simulink model "winter_simulink_IMM_control_2states"  (R2022a)
settings: Solver=FixedStepAuto  StartTime=0  StopTime=stop_time  FixedStep=simulation.time_step_H
values from neighbouring files (symbols this model uses):
  B_eq = param{6}    [measurement.m]    (also in measurement_2states.m; measurement_2states_3mes.m; measurement_3measure.m)
  rho = param{2}    [measurement_3measure.m]
undefined symbols (not defined in the file or in its folder): blade, dt, Gc, gearbox, generator, I_eq, IMM, lambda_vector, lookup_cP, omega_rated, pitch_range, pitch_vector, rotor, simulation, stop_time, T_R0, wind
libraries: simulink x2
settings Model: Creator=Niccolò  LastModifiedBy=Niccolò
settings SolverCC: ZeroCrossAlgorithm=Adaptive
settings DebuggingCC: IgnoredZcDiagnostic=none

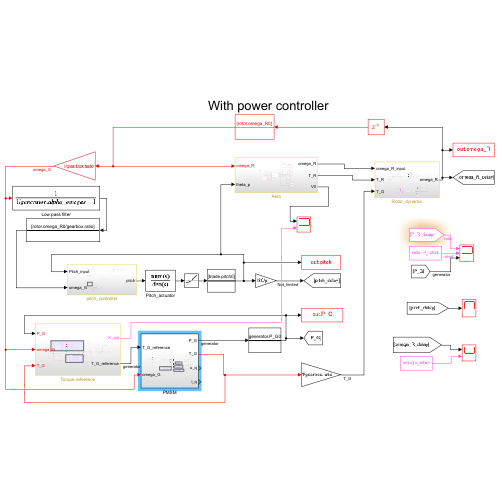
[thumbnail: Simulink's stored preview of the top-level diagram]
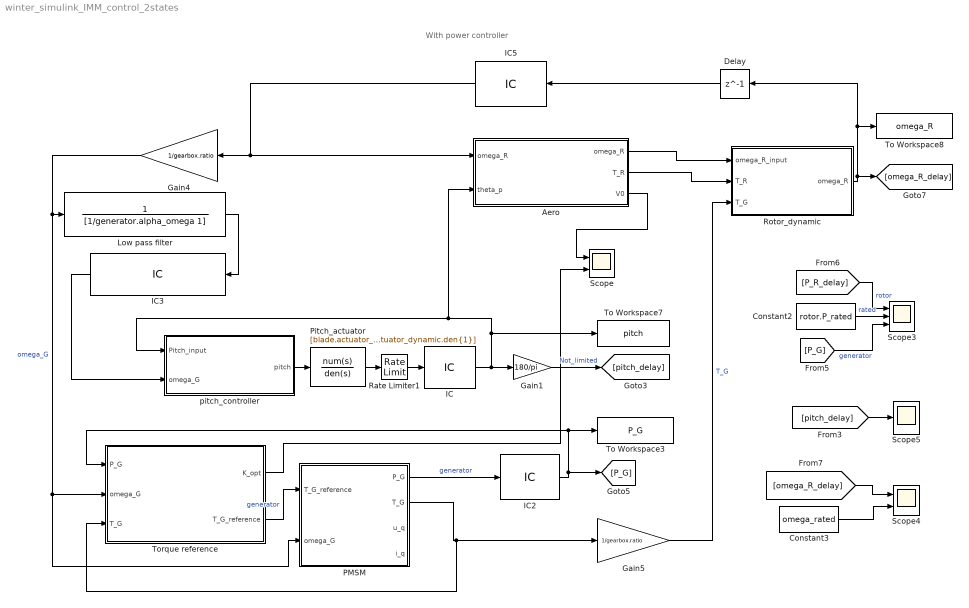
== system winter_simulink_IMM_control_2states ==
  note: With power controller
  Aero : Subsystem
  Constant2 : Constant  Value=rotor.P_rated
  Constant3 : Constant  Value=omega_rated
  Delay : Delay  DelayLength=1  InitialCondition=rotor.omega_R0
  Gain1 : Gain  Gain=180/pi
  Gain4 : Gain  Gain=1/gearbox.ratio
  Gain5 : Gain  Gain=1/gearbox.ratio
  IC : InitialCondition  Value=blade.pitch0
  IC2 : InitialCondition  Value=generator.P_G0
  IC3 : InitialCondition  Value=rotor.omega_R0/gearbox.ratio
  IC5 : InitialCondition  Value=rotor.omega_R0
  Low pass filter : TransferFcn  Denominator=[1/generator.alpha_omega 1]
  PMSM : Subsystem
  Pitch_actuator : TransferFcn  Numerator=[blade.actuator_dynamic.num{1}]  Denominator=[blade.actuator_dynamic.den{1}]
  Rate Limiter1 : RateLimiter  RisingSlewLimit=blade.pitch_rate  FallingSlewLimit=-blade.pitch_rate  SampleTimeMode=inherited
  Rotor_dynamic : Subsystem
  Scope : Scope  NumInputPorts=2
  Scope3 : Scope  NumInputPorts=3
  Scope4 : Scope  NumInputPorts=2
  Scope5 : Scope
  To Workspace3 : ToWorkspace  VariableName=P_G  SaveFormat=Timeseries  SampleTime=-1
  To Workspace7 : ToWorkspace  VariableName=pitch  SaveFormat=Timeseries  SampleTime=-1
  To Workspace8 : ToWorkspace  VariableName=omega_R  SaveFormat=Timeseries  SampleTime=-1
  Torque reference : Subsystem
  pitch_controller : Subsystem
  wires:
  [pitch_delay] -> Scope5/1
  Gain4/1 -> Low pass filter/1, PMSM/2(omega_G), Torque reference/2(omega_G)  "omega_G"
  Rate Limiter1/1 -> IC/1
  [P_R_delay] -> Scope3/1  "rotor"
  Constant3/1 -> Scope4/2
  Constant2/1 -> Scope3/2  "rated"
  [omega_R_delay] -> Scope4/1
  Gain1/1 -> [pitch_delay]  "Not_limited"
  [P_G] -> Scope3/3  "generator"
  Torque reference/2(T_G_reference) -> PMSM/1(T_G_reference)  "generator"
  pitch_controller/1(pitch) -> Pitch_actuator/1
  Pitch_actuator/1 -> Rate Limiter1/1
  Gain5/1 -> Rotor_dynamic/3(T_G)  "T_G"
  IC/1 -> Gain1/1, To Workspace7/1, pitch_controller/1(Pitch_input), Aero/2(theta_p)
  IC3/1 -> pitch_controller/2(omega_G)
  Rotor_dynamic/1(omega_R) -> Delay/1, To Workspace8/1, [omega_R_delay]
  IC5/1 -> Aero/1("omega_R "), Gain4/1
  IC2/1 -> [P_G], Torque reference/1(P_G), To Workspace3/1
  Aero/1(omega_R) -> Rotor_dynamic/1(omega_R_input)
  Aero/2(T_R) -> Rotor_dynamic/2(T_R)
  Low pass filter/1 -> IC3/1
  Delay/1 -> IC5/1
  Aero/3(V0) -> Scope/1
  Torque reference/1(K_opt) -> Scope/2
  PMSM/2(T_G) -> Torque reference/3(T_G), Gain5/1
  PMSM/1(P_G) -> IC2/1  "generator"

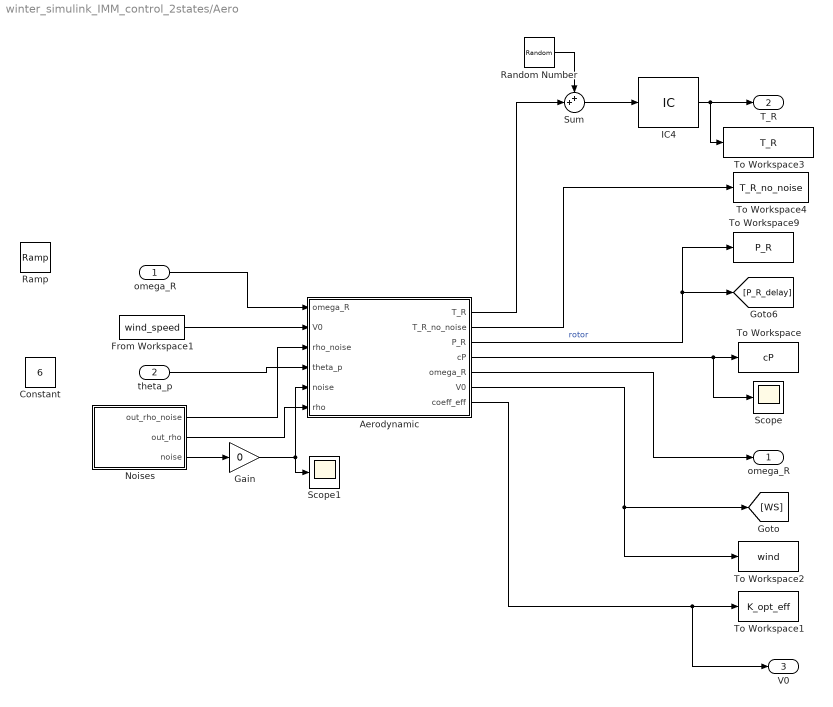
== system winter_simulink_IMM_control_2states/Aero ==
  "omega_R " : Inport
  theta_p : Inport  Port=2
  Aerodynamic : MATLAB Function  TreatAsAtomicUnit=on
  Constant : Constant  Value=6
  From Workspace1 : FromWorkspace  VariableName=wind_speed  SampleTime=1/wind.sample_f
  Gain : Gain  Gain=0
  IC4 : InitialCondition  Value=T_R0
  Noises : Subsystem
  Ramp : simulink/Sources/Ramp  slope=2/(stop_time-100)  start=100  InitialOutput=6
  Random Number : RandomNumber  Variance=IMM.Q(1)  SampleTime=simulation.time_step_H
  Scope : Scope
  Scope1 : Scope
  Sum : Sum  Inputs=++|
  To Workspace : ToWorkspace  VariableName=cP  SaveFormat=Timeseries  SampleTime=-1
  To Workspace1 : ToWorkspace  VariableName=K_opt_eff  SaveFormat=Timeseries  SampleTime=-1
  To Workspace2 : ToWorkspace  VariableName=wind  SaveFormat=Timeseries  SampleTime=-1
  To Workspace3 : ToWorkspace  VariableName=T_R  SaveFormat=Timeseries  SampleTime=-1
  To Workspace4 : ToWorkspace  VariableName=T_R_no_noise  SaveFormat=Timeseries  SampleTime=-1
  To Workspace9 : ToWorkspace  VariableName=P_R  SaveFormat=Timeseries  SampleTime=-1
  omega_R : Outport
  T_R : Outport  Port=2
  V0 : Outport  Port=3
  wires:
  "omega_R "/1 -> Aerodynamic/1("omega_R ")
  theta_p/1 -> Aerodynamic/4(theta_p)
  Aerodynamic/7(coeff_eff) -> V0/1, To Workspace1/1
  IC4/1 -> To Workspace3/1, T_R/1
  From Workspace1/1 -> Aerodynamic/2("V0 ")
  Aerodynamic/1(T_R) -> Sum/2
  Aerodynamic/2(T_R_no_noise) -> To Workspace4/1
  Aerodynamic/4(cP) -> Scope/1, To Workspace/1
  Aerodynamic/6(V0) -> To Workspace2/1, [WS]
  Aerodynamic/3(P_R) -> [P_R_delay], To Workspace9/1  "rotor"
  Noises/3(noise) -> Gain/1
  Gain/1 -> Aerodynamic/5(noise), Scope1/1
  Random Number/1 -> Sum/1
  Aerodynamic/5(omega_R) -> omega_R/1
  Sum/1 -> IC4/1
  Noises/1(out_rho_noise) -> Aerodynamic/3(rho_noise)
  Noises/2(out_rho) -> Aerodynamic/6(rho)

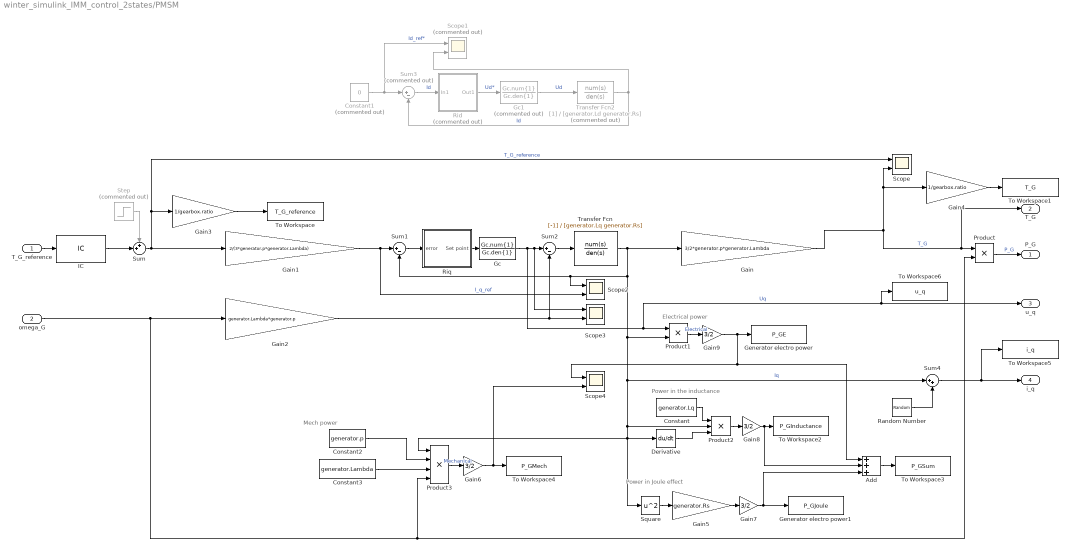
== system winter_simulink_IMM_control_2states/PMSM ==
  note: Power in Joule effect
  note: Power in the inductance
  note: Electrical power
  note: Mech power
  T_G_reference : Inport
  omega_G : Inport  Port=2
  Add : Sum  Inputs=3
  Constant : Constant  Value=generator.Lq
  Constant1 : Constant  Commented=on  Value=0
  Constant2 : Constant  Value=generator.p
  Constant3 : Constant  Value=generator.Lambda
  Derivative : Derivative
  Gain : Gain  Gain=3/2*generator.p*generator.Lambda
  Gain1 : Gain  Gain=2/(3*generator.p*generator.Lambda)
  Gain2 : Gain  Gain=generator.Lambda*generator.p
  Gain3 : Gain  Gain=1/gearbox.ratio
  Gain4 : Gain  Gain=1/gearbox.ratio
  Gain5 : Gain  Gain=generator.Rs
  Gain{6..9} (4 alike) : Gain  Gain=3/2
  Gc : TransferFcn  Numerator=Gc.num{1}  Denominator=Gc.den{1}
  Gc1 : TransferFcn  Commented=on  Numerator=Gc.num{1}  Denominator=Gc.den{1}
  Generator electro power : ToWorkspace  VariableName=P_GE  SaveFormat=Timeseries  SampleTime=-1
  Generator electro power1 : ToWorkspace  VariableName=P_GJoule  SaveFormat=Timeseries  SampleTime=-1
  IC : InitialCondition  Value=generator.T_G0
  Product : Product
  Product1 : Product
  Product2 : Product  Inputs=3
  Product3 : Product  Inputs=4
  Random Number : RandomNumber  Variance=IMM.Q(2,2)  SampleTime=simulation.time_step_H
  Rid : Subsystem  Commented=on
  Riq : Subsystem
  Scope{,2..4} (4 alike) : Scope  NumInputPorts=2
  Scope1 : Scope  Commented=on  NumInputPorts=2
  Square : Math  Operator=square
  Step : Step  Commented=on  Time=0.5  SampleTime=0
  Sum : Sum  Inputs=++|
  Sum1 : Sum  Inputs=|+-
  Sum2 : Sum  Inputs=|+-
  Sum3 : Sum  Commented=on  Inputs=|+-
  Sum4 : Sum  Inputs=|++
  To Workspace : ToWorkspace  VariableName=T_G_reference  SaveFormat=Timeseries  SampleTime=-1
  To Workspace1 : ToWorkspace  VariableName=T_G  SaveFormat=Timeseries  SampleTime=-1
  To Workspace2 : ToWorkspace  VariableName=P_GInductance  SaveFormat=Timeseries  SampleTime=-1
  To Workspace3 : ToWorkspace  VariableName=P_GSum  SaveFormat=Timeseries  SampleTime=-1
  To Workspace4 : ToWorkspace  VariableName=P_GMech  SaveFormat=Timeseries  SampleTime=-1
  To Workspace5 : ToWorkspace  VariableName=i_q  SaveFormat=Timeseries  SampleTime=-1
  To Workspace6 : ToWorkspace  VariableName=u_q  SaveFormat=Timeseries  SampleTime=-1
  Transfer Fcn : TransferFcn  Numerator=[-1]  Denominator=[generator.Lq generator.Rs]
  Transfer Fcn2 : TransferFcn  Commented=on  Denominator=[generator.Ld generator.Rs]
  P_G : Outport
  T_G : Outport  Port=2
  u_q : Outport  Port=3
  i_q : Outport  Port=4
  wires:
  Gc/1 -> To Workspace6/1, u_q/1, Product1/1, Scope3/1, Sum2/1  "Uq"
  Gain/1 -> T_G/1, Product/1, Gain4/1, Scope/2  "T_G"
  Riq/1(Set point) -> Gc/1
  Sum1/1 -> Riq/1(error)
  Transfer Fcn/1 -> Gain/1, Scope2/1, Sum1/2, Product1/2, Sum4/1, Product3/1, Square/1, Derivative/1, Product2/2  "Iq"
  Product/1 -> P_G/1  "P_G"
  Gain1/1 -> Scope2/2, Sum1/1  "I_q_ref"
  Sum/1 -> Gain1/1, Scope/1, Gain3/1  "T_G_reference"
  T_G_reference/1 -> IC/1
  Step/1 -> Sum/1
  Sum2/1 -> Transfer Fcn/1
  Gain3/1 -> To Workspace/1
  IC/1 -> Sum/2
  Gain5/1 -> Gain7/1
  Square/1 -> Gain5/1
  Derivative/1 -> Product2/3
  Constant/1 -> Product2/1
  Product2/1 -> Gain8/1
  Gc1/1 -> Transfer Fcn2/1  "Ud"
  Rid/1(Out1) -> Gc1/1  "Ud*"
  Transfer Fcn2/1 -> Sum3/2, Scope1/2  "Id"
  Constant1/1 -> Scope1/1, Sum3/1  "Id_ref*"
  Sum3/1 -> Rid/1(In1)  "Id"
  Add/1 -> To Workspace3/1
  Constant2/1 -> Product3/2
  Constant3/1 -> Product3/3
  Product3/1 -> Gain6/1  "Mechanical"
  Product1/1 -> Gain9/1  "Electrical"
  Gain2/1 -> Scope3/2, Sum2/2
  omega_G/1 -> Product/2, Product3/4, Gain2/1
  Gain6/1 -> Scope4/2, To Workspace4/1
  Gain7/1 -> Generator electro power1/1, Add/3
  Gain8/1 -> To Workspace2/1, Add/2
  Gain9/1 -> Generator electro power/1, Add/1, Scope4/1
  Gain4/1 -> To Workspace1/1
  Sum4/1 -> i_q/1, To Workspace5/1
  Random Number/1 -> Sum4/2

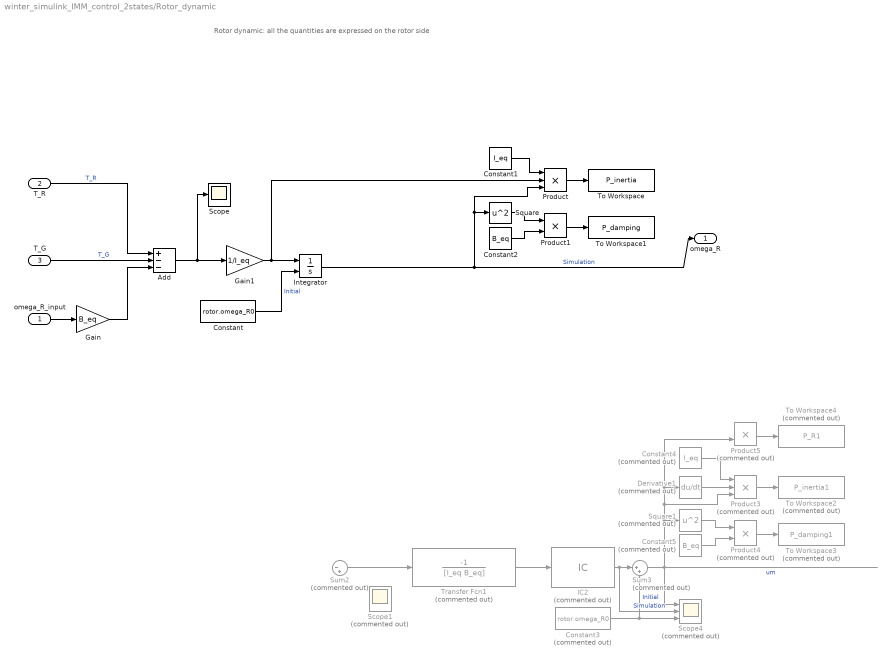
== system winter_simulink_IMM_control_2states/Rotor_dynamic ==
  note: Rotor dynamic: all the quantities are expressed on the rotor side
  omega_R_input : Inport
  T_R : Inport  Port=2
  T_G : Inport  Port=3
  Add : Sum  Inputs=+--
  Constant : Constant  Value=rotor.omega_R0
  Constant1 : Constant  Value=I_eq
  Constant2 : Constant  Value=B_eq
  Constant3 : Constant  Commented=on  Value=rotor.omega_R0
  Constant4 : Constant  Commented=on  Value=I_eq
  Constant5 : Constant  Commented=on  Value=B_eq
  Derivative1 : Derivative  Commented=on
  Gain : Gain  Gain=B_eq
  Gain1 : Gain  Gain=1/I_eq
  IC2 : InitialCondition  Commented=on  Value=rotor.omega_R0
  Integrator : Integrator  InitialConditionSource=external
  Product : Product  Inputs=3
  Product1 : Product
  Product3 : Product  Commented=on  Inputs=3
  Product4 : Product  Commented=on
  Product5 : Product  Commented=on
  Scope : Scope
  Scope1 : Scope  Commented=on  NumInputPorts=2
  Scope4 : Scope  Commented=on  NumInputPorts=3
  Square : Math  Operator=square
  Square1 : Math  Commented=on  Operator=square
  Sum2 : Sum  Commented=on  Inputs=|-+
  Sum3 : Sum  Commented=on  Inputs=|++
  To Workspace : ToWorkspace  VariableName=P_inertia  SaveFormat=Timeseries  SampleTime=-1
  To Workspace1 : ToWorkspace  VariableName=P_damping  SaveFormat=Timeseries  SampleTime=-1
  To Workspace2 : ToWorkspace  Commented=on  VariableName=P_inertia1  SaveFormat=Timeseries  SampleTime=-1
  To Workspace3 : ToWorkspace  Commented=on  VariableName=P_damping1  SaveFormat=Timeseries  SampleTime=-1
  To Workspace4 : ToWorkspace  Commented=on  VariableName=P_R1  SaveFormat=Timeseries  SampleTime=-1
  Transfer Fcn1 : TransferFcn  Commented=on  Numerator=[-1]  Denominator=[I_eq B_eq]
  omega_R : Outport
  wires:
  Integrator/1 -> Product/3, Square/1, omega_R/1  "Simulation"
  T_G/1 -> Add/2  "T_G"
  Constant/1 -> Integrator/2  "Initial"
  T_R/1 -> Add/1  "T_R"
  Add/1 -> Scope/1, Gain1/1
  Constant1/1 -> Product/1
  Product/1 -> To Workspace/1
  Constant2/1 -> Product1/2
  Product1/1 -> To Workspace1/1
  Square/1 -> Product1/1
  Square1/1 -> Product4/1
  Product5/1 -> To Workspace4/1
  Derivative1/1 -> Product3/2
  Product4/1 -> To Workspace3/1
  Constant4/1 -> Product3/1
  Constant5/1 -> Product4/2
  ? -> Scope1/2, Sum2/1, Product5/1  "T_R"
  ? -> Scope1/1, Sum2/2  "T_G"
  IC2/1 -> Scope4/2, Sum3/1  "Simulation"
  Sum2/1 -> Transfer Fcn1/1
  Product3/1 -> To Workspace2/1
  Transfer Fcn1/1 -> IC2/1
  Sum3/1 -> Product5/2, Derivative1/1, Product3/3, Square1/1, Scope4/1  "um"
  Constant3/1 -> Scope4/3, Sum3/2  "Initial"
  omega_R_input/1 -> Gain/1
  Gain/1 -> Add/3
  Gain1/1 -> Product/2, Integrator/1

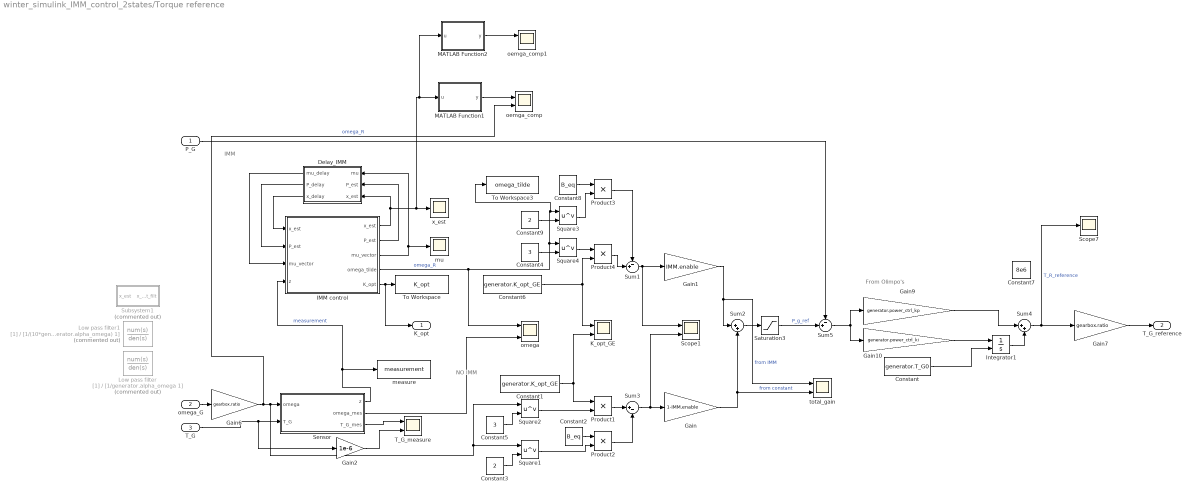
== system winter_simulink_IMM_control_2states/Torque reference ==
  note: IMM
  note: NO IMM
  note: From Olimpo's
  P_G : Inport
  omega_G : Inport  Port=2
  T_G : Inport  Port=3
  Constant : Constant  Value=generator.T_G0
  Constant1 : Constant  Value=generator.K_opt_GE
  Constant2 : Constant  Value=B_eq
  Constant3 : Constant  Value=2
  Constant4 : Constant  Value=3
  Constant5 : Constant  Value=3
  Constant6 : Constant  Value=generator.K_opt_GE
  Constant7 : Constant  Value=8e6
  Constant8 : Constant  Value=B_eq
  Constant9 : Constant  Value=2
  Delay_IMM : Subsystem
  Gain : Gain  Gain=1-IMM.enable
  Gain1 : Gain  Gain=IMM.enable
  Gain10 : Gain  Gain=generator.power_ctrl_ki
  Gain2 : Gain  Gain=1e-6
  Gain6 : Gain  Gain=gearbox.ratio
  Gain7 : Gain  Gain=gearbox.ratio
  Gain9 : Gain  Gain=generator.power_ctrl_kp
  IMM control : MATLAB Function  TreatAsAtomicUnit=on
  Integrator1 : Integrator  InitialConditionSource=external
  K_opt_GE : Scope  NumInputPorts=2
  Low pass filter : TransferFcn  Commented=on  Denominator=[1/generator.alpha_omega 1]
  Low pass filter1 : TransferFcn  Commented=on  Denominator=[1/(10*generator.alpha_omega) 1]
  MATLAB Function1 : MATLAB Function  TreatAsAtomicUnit=on
  MATLAB Function2 : MATLAB Function  TreatAsAtomicUnit=on
  Product{1..4} (4 alike) : Product
  Saturation3 : Saturate  UpperLimit=generator.P_rated  LowerLimit=0
  Scope1 : Scope  NumInputPorts=2
  Scope7 : Scope
  Sensor : MATLAB Function  TreatAsAtomicUnit=on
  Square{1..4} (4 alike) : Math  Operator=pow
  Subsystem1 : Subsystem  Commented=on
  Sum1 : Sum  Inputs=-+|
  Sum2 : Sum  Inputs=|++
  Sum3 : Sum  Inputs=|+-
  Sum4 : Sum  Inputs=|++
  Sum5 : Sum  Inputs=-+|
  T_G_measure : Scope  NumInputPorts=2
  To Workspace : ToWorkspace  VariableName=K_opt  SaveFormat=Timeseries  SampleTime=-1
  To Workspace3 : ToWorkspace  VariableName=omega_tilde  SaveFormat=Timeseries  SampleTime=-1
  measure : ToWorkspace  VariableName=measurement  SaveFormat=Timeseries  SampleTime=-1
  mu : Scope
  oemga_comp : Scope  NumInputPorts=2
  oemga_comp1 : Scope  NumInputPorts=2
  omega : Scope  NumInputPorts=3
  total_gain : Scope  NumInputPorts=2
  x_est : Scope
  K_opt : Outport
  T_G_reference : Outport  Port=2
  wires:
  Square2/1 -> Product1/2
  Gain9/1 -> Sum4/1
  Gain10/1 -> Integrator1/1
  Constant/1 -> Integrator1/2
  Sum4/1 -> Scope7/1, Gain7/1  "T_R_reference"
  Constant5/1 -> Square2/2
  Saturation3/1 -> Sum5/2  "P_g_ref"
  Integrator1/1 -> Sum4/2
  Sum5/1 -> Gain9/1, Gain10/1
  Gain7/1 -> T_G_reference/1
  P_G/1 -> Sum5/1
  IMM control/2(P_est) -> Delay_IMM/2(P_est)
  Delay_IMM/3(x_delay) -> IMM control/1("x_est ")
  Delay_IMM/2(P_delay) -> IMM control/2("P_est ")
  Delay_IMM/1(mu_delay) -> IMM control/3("mu_vector ")
  IMM control/3(mu_vector) -> Delay_IMM/1(mu), mu/1
  Constant8/1 -> Product3/1
  Square3/1 -> Product3/2
  Product4/1 -> Sum1/2
  Sum1/1 -> Scope1/1, Gain1/1
  Constant9/1 -> Square3/2
  Gain/1 -> total_gain/2, Sum2/2  "from constant"
  Sum2/1 -> Saturation3/1
  Constant3/1 -> Square1/2
  Sum3/1 -> Scope1/2, Gain/1
  Product1/1 -> Sum3/1
  Square1/1 -> Product2/2
  Product2/1 -> Sum3/2
  Constant2/1 -> Product2/1
  Gain1/1 -> total_gain/1, Sum2/1  "from IMM"
  Square4/1 -> Product4/1
  Product3/1 -> Sum1/1
  Constant1/1 -> Product1/1, K_opt_GE/2
  IMM control/5(K_opt) -> K_opt/1, To Workspace/1
  Constant4/1 -> Square4/2
  omega_G/1 -> Gain6/1
  Constant6/1 -> K_opt_GE/1, Product4/2
  Sensor/1(z) -> measure/1, IMM control/4(z)  "measurement"
  MATLAB Function1/1(y) -> oemga_comp/1
  Gain6/1 -> Square2/1, Square1/1, Sensor/1(omega), oemga_comp/2  "omega_R"
  T_G/1 -> Gain2/1, Sensor/2(T_G)
  IMM control/4(omega_tilde) -> To Workspace3/1, Square3/1, Square4/1, omega/1  "omega_R"
  Sensor/3(T_G_mes) -> T_G_measure/1
  Gain2/1 -> T_G_measure/2
  Sensor/2(omega_mes) -> omega/3
  IMM control/1(x_est) -> MATLAB Function2/1(u), MATLAB Function1/1(u), x_est/1, Delay_IMM/3(x_est)
  MATLAB Function2/1(y) -> oemga_comp1/1
  ? -> oemga_comp1/2  "omega_R"

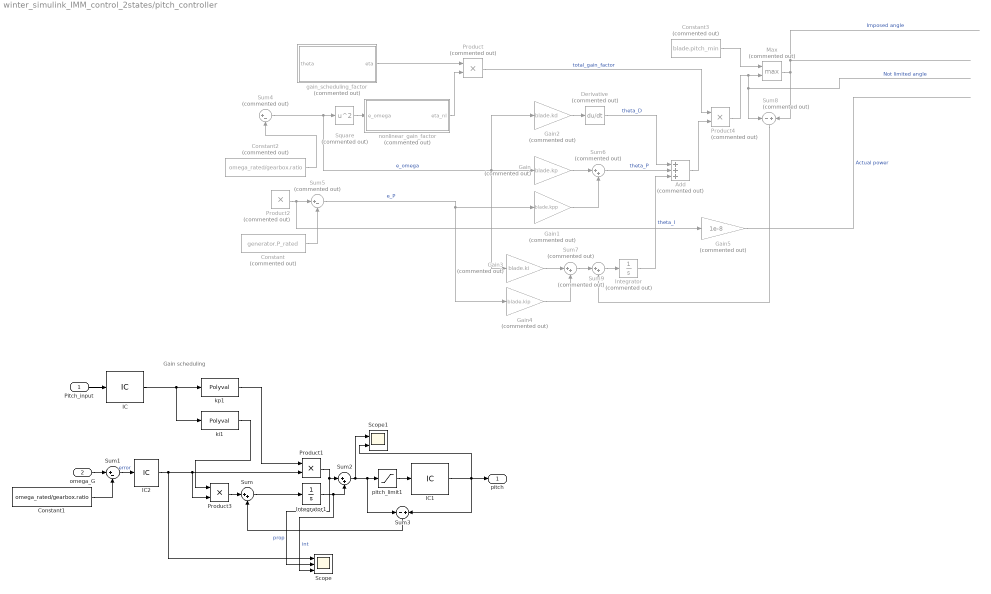
== system winter_simulink_IMM_control_2states/pitch_controller ==
  note: Gain scheduling
  Pitch_input : Inport
  omega_G : Inport  Port=2
  Add : Sum  Commented=on  Inputs=+++
  Constant : Constant  Commented=on  Value=generator.P_rated
  Constant1 : Constant  Value=omega_rated/gearbox.ratio
  Constant2 : Constant  Commented=on  Value=omega_rated/gearbox.ratio
  Constant3 : Constant  Commented=on  Value=blade.pitch_min
  Derivative : Derivative  Commented=on
  Gain : Gain  Commented=on  Gain=blade.kp
  Gain1 : Gain  Commented=on  Gain=blade.kpp
  Gain2 : Gain  Commented=on  Gain=blade.kd
  Gain3 : Gain  Commented=on  Gain=blade.ki
  Gain4 : Gain  Commented=on  Gain=blade.kip
  Gain5 : Gain  Commented=on  Gain=1e-8
  IC : InitialCondition  Value=blade.pitch0
  IC1 : InitialCondition  Value=blade.pitch0
  IC2 : InitialCondition  Value=(rotor.omega_R0 - omega_rated)/gearbox.ratio
  Integrator : Integrator  Commented=on
  Integrator1 : Integrator
  Max : MinMax  Commented=on  Function=max  Inputs=2
  Product : Product  Commented=on
  Product1 : Product
  Product2 : Product  Commented=on
  Product3 : Product
  Product4 : Product  Commented=on
  Scope : Scope  NumInputPorts=3
  Scope1 : Scope  NumInputPorts=2
  Square : Math  Commented=on  Operator=square
  Sum : Sum  Inputs=|++
  Sum1 : Sum  Inputs=|+-
  Sum2 : Sum  Inputs=|++
  Sum3 : Sum  Inputs=-|+
  Sum4 : Sum  Commented=on  Inputs=|+-
  Sum5 : Sum  Commented=on  Inputs=|+-
  Sum6 : Sum  Commented=on  Inputs=|++
  Sum7 : Sum  Commented=on  Inputs=|++
  Sum8 : Sum  Commented=on  Inputs=-|+
  Sum9 : Sum  Commented=on  Inputs=|++
  gain_scheduling_factor : MATLAB Function  Commented=on  TreatAsAtomicUnit=on
  ki1 : Polyval  Coefs=blade.ki_schedule
  kp1 : Polyval  Coefs=blade.kp_schedule
  nonlinear_gain_factor : MATLAB Function  Commented=on  TreatAsAtomicUnit=on
  pitch_limit1 : Saturate  UpperLimit=pitch_range(2)  LowerLimit=0
  pitch : Outport
  wires:
  Sum/1 -> Integrator1/1
  Constant1/1 -> Sum1/2
  Product3/1 -> Sum/1
  omega_G/1 -> Sum1/1
  ki1/1 -> Product3/1
  kp1/1 -> Product1/1
  Sum1/1 -> IC2/1  "error"
  Product1/1 -> Scope/2, Sum2/1  "prop"
  Integrator1/1 -> Scope/3, Sum2/2  "int"
  ? -> ?  "Actual value"
  Sum8/1 -> Sum9/2
  Product4/1 -> Max/2, Sum8/1  "Not limited angle"
  Add/1 -> Product4/2
  Gain4/1 -> Sum7/2
  Product2/1 -> Gain5/1, Sum5/1
  Integrator/1 -> Add/3  "theta_I"
  ? -> Product2/2
  Derivative/1 -> Add/1  "theta_D"
  Product/1 -> Product4/1  "total_gain_factor"
  Sum6/1 -> Add/2  "theta_P"
  nonlinear_gain_factor/1(eta_nl) -> Product/2
  gain_scheduling_factor/1(eta) -> Product/1
  Gain/1 -> Sum6/1
  Max/1 -> Sum8/2  "Imposed angle"
  Sum5/1 -> Gain4/1, Gain1/1  "e_P"
  ? -> Sum4/1, Product2/1
  Constant2/1 -> Sum4/2
  Sum4/1 -> Gain3/1, Gain2/1, Gain/1, Square/1  "e_omega"
  Gain2/1 -> Derivative/1
  ? -> gain_scheduling_factor/1(theta)
  Gain5/1 -> ?  "Actual power"
  Constant/1 -> Sum5/2
  Constant3/1 -> Max/1
  Sum9/1 -> Integrator/1
  Gain1/1 -> Sum6/2
  Sum7/1 -> Sum9/1
  Square/1 -> nonlinear_gain_factor/1(e_omega)
  Gain3/1 -> Sum7/1
  Pitch_input/1 -> IC/1
  Sum2/1 -> pitch_limit1/1, Sum3/1, Scope1/1
  Sum3/1 -> Sum/2
  pitch_limit1/1 -> IC1/1
  IC/1 -> ki1/1, kp1/1
  IC1/1 -> Scope1/2, pitch/1, Sum3/2
  IC2/1 -> Scope/1, Product3/2, Product1/2

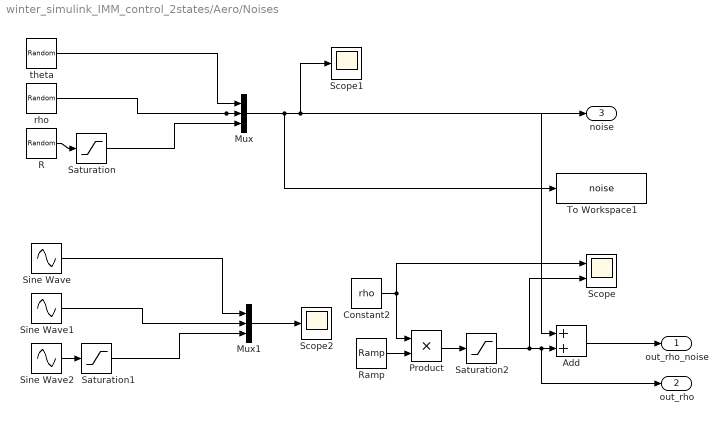
== system winter_simulink_IMM_control_2states/Aero/Noises ==
  Add : Sum
  Constant2 : Constant  Value=rho
  Mux : Mux  Inputs=3
  Mux1 : Mux  Inputs=3
  Product : Product
  R : RandomNumber  Variance=(IMM.sigma_R)^2  SampleTime=simulation.time_step_H
  Ramp : simulink/Sources/Ramp  slope=0.4/(stop_time-50)  start=50  InitialOutput=0.8
  Saturation : Saturate  UpperLimit=0  LowerLimit=-10
  Saturation1 : Saturate  UpperLimit=0  LowerLimit=-10
  Saturation2 : Saturate  UpperLimit=1.2*rho
  Scope : Scope  NumInputPorts=2
  Scope1 : Scope
  Scope2 : Scope
  Sine Wave : Sin  Amplitude=IMM.sigma_theta  Frequency=IMM.freq_theta  Phase=IMM.phase_theta  SampleTime=simulation.time_step_H
  Sine Wave1 : Sin  Amplitude=IMM.sigma_rho  Frequency=IMM.freq_rho  Phase=IMM.phase_rho  SampleTime=simulation.time_step_H
  Sine Wave2 : Sin  Amplitude=IMM.sigma_R  Frequency=IMM.freq_R  Phase=IMM.phase_R  SampleTime=simulation.time_step_H
  To Workspace1 : ToWorkspace  VariableName=noise  SaveFormat=Timeseries  SampleTime=-1
  rho : RandomNumber  Variance=(IMM.sigma_rho)^2  SampleTime=simulation.time_step_H
  theta : RandomNumber  Variance=(IMM.sigma_theta)^2  SampleTime=simulation.time_step_H
  out_rho_noise : Outport
  out_rho : Outport  Port=2
  noise : Outport  Port=3
  wires:
  Mux/1 -> To Workspace1/1, noise/1, Scope1/1
  theta/1 -> Mux/1
  rho/1 -> Add/1, Mux/2
  Saturation/1 -> Mux/3
  R/1 -> Saturation/1
  Mux1/1 -> Scope2/1
  Sine Wave2/1 -> Saturation1/1
  Sine Wave/1 -> Mux1/1
  Saturation1/1 -> Mux1/3
  Sine Wave1/1 -> Mux1/2
  Constant2/1 -> Product/1, Scope/1
  Product/1 -> Saturation2/1
  Add/1 -> out_rho_noise/1
  Saturation2/1 -> Scope/2, out_rho/1, Add/2
  Ramp/1 -> Product/2

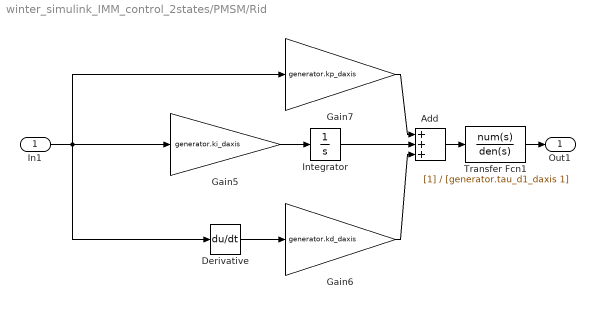
== system winter_simulink_IMM_control_2states/PMSM/Rid ==
  In1 : Inport
  Add : Sum  Inputs=+++
  Derivative : Derivative
  Gain5 : Gain  Gain=generator.ki_daxis
  Gain6 : Gain  Gain=generator.kd_daxis
  Gain7 : Gain  Gain=generator.kp_daxis
  Integrator : Integrator
  Transfer Fcn1 : TransferFcn  Denominator=[generator.tau_d1_daxis 1]
  Out1 : Outport
  wires:
  Integrator/1 -> Add/2
  Add/1 -> Transfer Fcn1/1
  Gain7/1 -> Add/1
  Gain6/1 -> Add/3
  Derivative/1 -> Gain6/1
  In1/1 -> Derivative/1, Gain7/1, Gain5/1
  Transfer Fcn1/1 -> Out1/1
  Gain5/1 -> Integrator/1

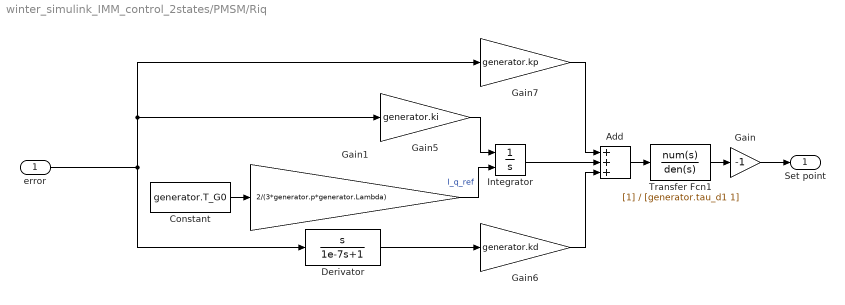
== system winter_simulink_IMM_control_2states/PMSM/Riq ==
  error : Inport
  Add : Sum  Inputs=+++
  Constant : Constant  Value=generator.T_G0
  Derivator : TransferFcn  Numerator=[1 0]  Denominator=[1e-7 1]
  Gain : Gain  Gain=-1
  Gain1 : Gain  Gain=2/(3*generator.p*generator.Lambda)
  Gain5 : Gain  Gain=generator.ki
  Gain6 : Gain  Gain=generator.kd
  Gain7 : Gain  Gain=generator.kp
  Integrator : Integrator  InitialConditionSource=external
  Transfer Fcn1 : TransferFcn  Denominator=[generator.tau_d1 1]
  Set point : Outport
  wires:
  Integrator/1 -> Add/2
  Add/1 -> Transfer Fcn1/1
  Constant/1 -> Gain1/1
  Gain7/1 -> Add/1
  Gain6/1 -> Add/3
  Derivator/1 -> Gain6/1
  Transfer Fcn1/1 -> Gain/1
  Gain5/1 -> Integrator/1
  Gain1/1 -> Integrator/2  "I_q_ref"
  Gain/1 -> Set point/1
  error/1 -> Gain5/1, Gain7/1, Derivator/1

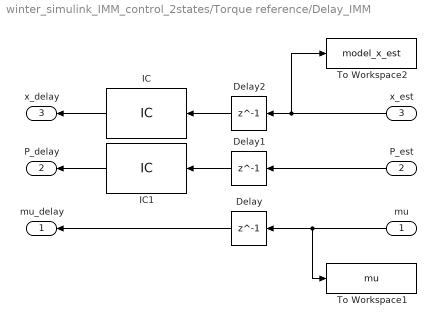
== system winter_simulink_IMM_control_2states/Torque reference/Delay_IMM ==
  mu : Inport
  P_est : Inport  Port=2
  x_est : Inport  Port=3
  Delay : Delay  DelayLength=1  InitialCondition=ones(IMM.n_models, 1)/IMM.n_models
  Delay1 : Delay  DelayLength=1  InitialCondition=IMM.P_est_initial
  Delay2 : Delay  DelayLength=1  InitialCondition=IMM.x_est_initial
  IC : InitialCondition  Value=IMM.x_est_initial
  IC1 : InitialCondition  Value=IMM.P_est_initial
  To Workspace1 : ToWorkspace  VariableName=mu  SaveFormat=Timeseries  SampleTime=-1
  To Workspace2 : ToWorkspace  VariableName=model_x_est  SaveFormat=Timeseries  SampleTime=-1
  mu_delay : Outport
  P_delay : Outport  Port=2
  x_delay : Outport  Port=3
  wires:
  Delay1/1 -> IC1/1
  P_est/1 -> Delay1/1
  Delay2/1 -> IC/1
  mu/1 -> To Workspace1/1, Delay/1
  x_est/1 -> To Workspace2/1, Delay2/1
  IC/1 -> x_delay/1
  IC1/1 -> P_delay/1
  Delay/1 -> mu_delay/1

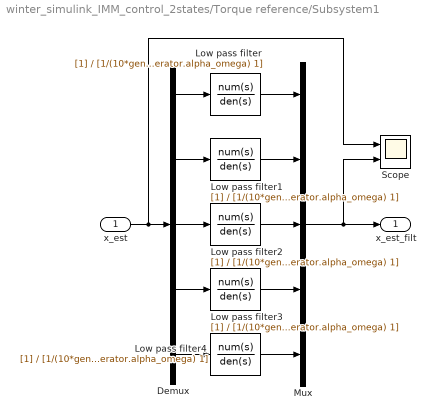
== system winter_simulink_IMM_control_2states/Torque reference/Subsystem1 ==
  x_est : Inport
  Demux : Demux  Outputs=5
  Low pass filter{,1..4} (5 alike) : TransferFcn  Denominator=[1/(10*generator.alpha_omega) 1]
  Mux : Mux  Inputs=5
  Scope : Scope  NumInputPorts=2
  x_est_filt : Outport
  wires:
  Demux/3 -> Low pass filter2/1
  Demux/1 -> Low pass filter/1
  Demux/4 -> Low pass filter3/1
  x_est/1 -> Scope/1, Demux/1
  Demux/5 -> Low pass filter4/1
  Demux/2 -> Low pass filter1/1
  Low pass filter4/1 -> Mux/5
  Low pass filter3/1 -> Mux/4
  Low pass filter2/1 -> Mux/3
  Low pass filter1/1 -> Mux/2
  Low pass filter/1 -> Mux/1
  Mux/1 -> Scope/2, x_est_filt/1

== matlab function winter_simulink_IMM_control_2states/pitch_controller/gain_scheduling_factor ==
  data: eta output; theta input; blade parameter
function eta = gain_scheduling_factor(theta, blade)

K1 = blade.K1;
K2 = blade.K2;

theta = theta*180/pi; % [deg]

eta = 1/(1+ theta/K1 + theta^2/K2);

== matlab function winter_simulink_IMM_control_2states/pitch_controller/nonlinear_gain_factor ==
  data: e_omega input; eta_nl output; blade parameter; generator parameter
function eta_nl = nonlinear_gain_factor(e_omega, blade, generator)

omega_rated = generator.omega_rated;
omega2 = omega_rated*blade.omega2omega0ratio;

eta_nl = 1 + e_omega^2/(omega2 - omega_rated)^2;

== matlab function winter_simulink_IMM_control_2states/Torque reference/MATLAB Function1 ==
  data: u input; y output
function y = fcn(u)

y = u(1,:);

== matlab function winter_simulink_IMM_control_2states/Aero/Aerodynamic ==
  data: omega_R input; V0 input; T_R output; T_R_no_noise output; P_R output; rho_noise input; theta_p input; lambda_vector parameter; pitch_vector parameter; lookup_cP parameter; cP output; rotor parameter; omega_R output; V0 output; noise input; coeff_eff output; rho input
function [T_R, T_R_no_noise, P_R, cP, omega_R, V0, coeff_eff] = Aerodynamic(omega_R, V0, rho_noise, theta_p, lambda_vector, pitch_vector, lookup_cP, rotor, noise, rho)

R = rotor.R;       % rotor radius [m]

% retrive the cP from the look-up table
lambda = omega_R*R/V0;                                                
cP = interp2(lambda_vector, pitch_vector, lookup_cP, lambda, theta_p);

P_R = 0.5*rho*V0^3*pi*R^2*cP; % rotor power [W]
T_R_no_noise = P_R/omega_R;            % rotor torque [Nm]


theta_p = theta_p + noise(1); % pitch angle [rad]
R = rotor.R + noise(3);       % rotor radius [m]

% retrive the cP from the look-up table
lambda = omega_R*R/V0;                                                
cP = interp2(lambda_vector, pitch_vector, lookup_cP, lambda, theta_p);
P_R = 0.5*rho_noise*V0^3*pi*R^2*cP; % rotor power [W]
T_R = P_R/omega_R;            % rotor torque [Nm]

coeff_eff =cP*rho*R^2; %

== matlab function winter_simulink_IMM_control_2states/Torque reference/IMM control ==
  settings: updateMethod=DISCRETE  sampleTime=simulation.time_step_H
  data: x_est output; P_est output; mu_vector output; x_est input size=[IMM.states_len, IMM.n_models]; P_est input size=[IMM.states_len, IMM.states_len, IMM.n_models]; mu_vector input size=[IMM.n_models, 1]; IMM parameter; I_eq parameter; omega_tilde output size=1; K_opt output size=1; dt parameter; z input; generator parameter; B_eq parameter
function [x_est, P_est, mu_vector, omega_tilde,  K_opt] = gain_IMM(x_est, P_est, mu_vector, IMM, I_eq, dt, z, generator, B_eq)
  % x_est -> (states_len, n_models) items containing the state estimation
  % P_est -> (states_len, states_len, n_models) containing the covariance
  
  n_models = IMM.n_models; % number of models to test
  states_len = IMM.states_len; % length of the states
  measure_len = IMM.measure_len; % length of the measurement
  Pi = IMM.Pi; 
  R = IMM.W;
  Q = IMM.Q;
  K_vector = IMM.K_vector;
  mu = zeros(n_models);
  % Vector of parameters
  param = cell(6,1);
  param{1} = I_eq; % inertia
  param{2} = 0; % cp*rho*R^2
  param{3} = generator.K_opt_GE; % K_opt
  param{4} = R; % measure noise
  param{5} = Q; % process noise 
  param{6} = B_eq; % transmission damping
 
  % Assamble the model cell
  model = cell(n_models, 1);
  for j=1:n_models
    param{2} = IMM.K_vector(j); % rho_cp_R2
    model{j} = struct('rho_cp_R2', IMM.K_vector(j), 'x_est', x_est(1:states_len, j), 'P_est', P_est(1:states_len,1:states_len,j), 'z_hat', zeros(measure_len, 1), 'P_prior', P_est(1:states_len,1:states_len,j), 'Lambda', 0, 'mu', mu_vector(j), 'mu_new', 0, 'x_tilde', zeros(states_len, 1), 'P_tilde', zeros(states_len));
  end
  
  % Filtering
  u = [0]; % input
  model = filtering(model, z, u, param, dt);
  
  % Mode probability updating
  model = probability_updating(model, z, param, dt);
  K_opt = compute_K_opt(model); % weighted mean of the filters

  % State combination
  x_est_g = zeros(states_len, 1); % global state
  [x_est_g(1:states_len, 1), ~] = state_combination(model);
  omega_tilde = x_est_g(1); % estimation of the rotational speed

  % Filter interaction
  [model, model_prob] = filter_interaction(model, Pi);
  
  % Assemble the model cell
  for j=1:n_models
    x_est(1:states_len, j) = model{j}.x_est(1:states_len);
    P_est(1:states_len,1:states_len,j) = model{j}.P_est(1:states_len, 1:states_len);
    mu_vector(j) = model{j}.mu_new(1);
  end
  
end
  
  %   _____ _  _______ 
  %  | ____| |/ /  ___|
  %  |  _| | ' /| |_   
  %  | |___| . \|  _|  
  %  |_____|_|\_\_|    
                     
  function [model] = EKF(model, z, u, param, matrices, dt)
    % y -> measurement of the rotational speed [rad/s]
    
    x_est = model.x_est;
    P_est = model.P_est;
    states_len = size(x_est, 1);
    measure_len = size(z, 1);

    F = matrices.F;
    H = matrices.H;
    Q = matrices.Q;
    R = matrices.R;
    G = matrices.G;
  
    % Prediction
    x_est = dynamic(x_est(1:states_len), u, param, dt);
    P_est = F*P_est*F' + G*Q*G';
    P_prior = P_est;
    states_len = size(x_est, 1); % number of states
  
    % Update
    [~, z_hat] = measurement(x_est, param, measure_len); % estimation of the measurement using the sensor's model
    Innovation = z - z_hat;
    S_Inno = H*P_est*H' + R;
    W = P_est*H'*inv(S_Inno); % kalman gain
    x_est = x_est + W*Innovation; % update state estimate
    P_est = (eye(states_len) - W*H)*P_est; % update covariance matrix
  
  
    model.x_est(1:states_len) = x_est(1:states_len);
    model.P_est(1:states_len, 1:states_len) = P_est(1:states_len, 1:states_len);
    model.z_hat = z_hat;
    model.P_prior = P_prior;
  end
  
  %   ____                              _      
  %  |  _ \ _   _ _ __   __ _ _ __ ___ (_) ___ 
  %  | | | | | | | '_ \ / _` | '_ ` _ \| |/ __|
  %  | |_| | |_| | | | | (_| | | | | | | | (__ 
  %  |____/ \__, |_| |_|\__,_|_| |_| |_|_|\___|
  %         |___/                              
  
  function x_new = dynamic(x_est, u, param, dt)
  
    states_len = size(x_est, 1);
    I_eq = param{1}; % Inertia
    rho_cp_R2 = param{2}; % Damping
    K_opt = param{3}; % Power coefficient
    
    omega = x_est(1);
    V0 = x_est(2);

    x_new = zeros(states_len,1);
  
    x_new(1) = omega + dt/I_eq*(1/2*pi*rho_cp_R2*V0^3/omega - K_opt*omega^2 ); % [rad/s] rotational speed
    x_new(2) = V0; % [m/s] wind speed 
  end
  

  
  %    ____                            _                         _     
  %   / ___|___  _ __ ___  _ __  _   _| |_ ___   _ __ ___   __ _| |_   
  %  | |   / _ \| '_ ` _ \| '_ \| | | | __/ _ \ | '_ ` _ \ / _` | __|  
  %  | |__| (_) | | | | | | |_) | |_| | ||  __/ | | | | | | (_| | |_ _ 
  %   \____\___/|_| |_| |_| .__/ \__,_|\__\___| |_| |_| |_|\__,_|\__(_)
  %                       |_|                                          
  
  function matrices = compute_matrices(x_est, param, dt)
  
    I_eq = param{1}; % Inertia
    rho_cp_R2 = param{2}; % Density
    K_opt = param{3}; % Power coefficient
    B_eq = param{6};
    omega = x_est(1);
    V0 = x_est(2);

    F = [1+dt/I_eq*(-1/2*rho_cp_R2*pi*V0^3/omega^2-2*K_opt*omega), (3*dt*pi*rho_cp_R2*V0^2)/(2*I_eq*omega); 0, 1];
    H = [1, 0; (-1/2*pi*rho_cp_R2*V0^3/omega^2-B_eq)*1e-6, (3/2*pi*rho_cp_R2*V0^2/omega)*1e-6];
    G = [dt/I_eq 0; 0 1];

    matrices = struct('F', F, 'H', H, 'G', G);
  end
  
  %   _____ _ _ _            _             
  %  |  ___(_) | |_ ___ _ __(_)_ __   __ _ 
  %  | |_  | | | __/ _ \ '__| | '_ \ / _` |
  %  |  _| | | | ||  __/ |  | | | | | (_| |
  %  |_|   |_|_|\__\___|_|  |_|_| |_|\__, |
  %                                  |___/ 
  
  function model = filtering(model, z, u, param, dt)
    n_models = size(model, 1);
    states_len = size(model{1}.x_est, 1);
    for j=1:n_models
      param{2} = model{j}.rho_cp_R2;
      % compute the linearized matrices
      matrices = compute_matrices(model{j}.x_est(1:states_len), param, dt);
      matrices.R = param{4};
      matrices.Q = param{5};
  
      [model{j}] = EKF(model{j}, z, u, param, matrices, dt);
    end
  end
  
  %   ____            _                       _       _   _             
  %  |  _ \ _ __ ___ | |__    _   _ _ __   __| | __ _| |_(_)_ __   __ _ 
  %  | |_) | '__/ _ \| '_ \  | | | | '_ \ / _` |/ _` | __| | '_ \ / _` |
  %  |  __/| | | (_) | |_) | | |_| | |_) | (_| | (_| | |_| | | | | (_| |
  %  |_|   |_|  \___/|_.__/   \__,_| .__/ \__,_|\__,_|\__|_|_| |_|\__, |
  %                                |_|                            |___/ 
  
  function model = probability_updating(model, z, param, dt)
    n_models = size(model, 1);
    states_len = size(model{1}.x_est, 1);
    
    for j=1:n_models
      % compute the linearized matrices
      matrices = compute_matrices(model{j}.x_est(1:states_len), param, dt);
      matrices.R = param{4};
      matrices.Q = param{5}; 

      model{j}.Lambda = zeros(1);
      zeta = zeros(states_len, 1);

      H = matrices.H;
      R = matrices.R;
      G = matrices.G;
      z_hat = model{j}.z_hat;
      P_prior = model{j}.P_prior;
      
      S = zeros(states_len, states_len);
      S = H*P_prior*H' + R;
      zeta = z - z_hat;
%       tmp = 1/sqrt(2*pi*max(det(S), 1e-80))*exp(-1/2*zeta'*inv(S)*zeta);
%       tmp = max(tmp, 1e-80);
      tmp = 1/sqrt(2*pi*det(S))*exp(-1/2*zeta'*inv(S)*zeta);
      model{j}.Lambda = tmp(1);
    end
    % Compute the denominator
    den = 0;
    for j=1:n_models
      den = den + model{j}.mu*model{j}.Lambda;
    end
    % Update model probability
    for j=1:n_models
      model{j}.mu = model{j}.mu*model{j}.Lambda/den;
    end
  end
  
  %   ____  _        _                             _      
  %  / ___|| |_ __ _| |_ ___    ___ ___  _ __ ___ | |__   
  %  \___ \| __/ _` | __/ _ \  / __/ _ \| '_ ` _ \| '_ \  
  %   ___) | || (_| | ||  __/ | (_| (_) | | | | | | |_) | 
  %  |____/ \__\__,_|\__\___|  \___\___/|_| |_| |_|_.__(_)
                                                        
  function [x_est, P_est] = state_combination(model)
    n_models = size(model, 1);
    states_len = size(model{1}.x_est, 1);
    x_est = zeros(states_len,1);
    P_est = zeros(states_len,states_len);
    for j=1:n_models
      x_est(1:states_len) = x_est(1:states_len) + model{j}.mu*model{j}.x_est(1:states_len);
    end
    
    for j=1:n_models
      P_est = P_est + model{j}.mu*(model{j}.P_est + (x_est - model{j}.x_est)*(x_est - model{j}.x_est)');
    end
  
  end
  
  %   _____ _ _ _              _       _                      _   _             
  %  |  ___(_) | |_ ___ _ __  (_)_ __ | |_ ___ _ __ __ _  ___| |_(_) ___  _ __  
  %  | |_  | | | __/ _ \ '__| | | '_ \| __/ _ \ '__/ _` |/ __| __| |/ _ \| '_ \ 
  %  |  _| | | | ||  __/ |    | | | | | ||  __/ | | (_| | (__| |_| | (_) | | | |
  %  |_|   |_|_|\__\___|_|    |_|_| |_|\__\___|_|  \__,_|\___|\__|_|\___/|_| |_|
                                                                              
  function [model, model_prob] = filter_interaction(model, Pi)
    n_models = size(model, 1);
    states_len = size(model{1}.x_est, 1);
    mu = zeros(n_models, n_models);
  
    for j=1:n_models
      model{j}.mu_new = 0;
      for i=1:n_models
          model{j}.mu_new = model{j}.mu_new + Pi(i, j)*model{i}.mu; 
      end
    end
  
    for j=1:n_models
      for i=1:n_models
          mu(i, j) = Pi(i, j)*model{i}.mu/model{j}.mu_new;
      end
    end
  
    for j=1:n_models
      model{j}.x_tilde(1:states_len, 1) = zeros(states_len, 1);
      model{j}.P_tilde = zeros(states_len, states_len);
      for i=1:n_models
        model{j}.x_tilde = model{j}.x_tilde + mu(i, j)*model{i}.x_est;
      end
      for i=1:n_models
          model{j}.P_tilde = model{j}.P_tilde + mu(i, j)*(model{i}.P_est + (model{j}.x_tilde - model{i}.x_est)*(model{j}.x_tilde - model{i}.x_est)');
      end
      model{j}.x_est = model{j}.x_tilde;
      model{j}.P_est = model{j}.P_tilde;
    end
  
    % Store the value of the probability
    model_prob = zeros(n_models, 1);
    for j=1:n_models
      model_prob(j) = model{j}.mu_new;
    end
  end
  
  %                                       _ 
  %   _ __ _____   ___ __  _ __ _ __   __| |
  %  | '_ ` _ \ \ / / '_ \| '__| '_ \ / _` |
  %  | | | | | \ V /| | | | |  | | | | (_| |
  %  |_| |_| |_|\_/ |_| |_|_|  |_| |_|\__,_|
                                          
  function y = my_mvnrnd(mu, cov, n)
      % Cholesky decomposition
      L = chol(cov, 'lower');
  
      % Generate standard normal random numbers
      z = randn(n, length(mu));
  
      % Transform to multivariate normal
      y = L*z' + mu;
  
      y = y';
  end

  %    ___        _               _   
  %   / _ \ _   _| |_ _ __  _   _| |_ 
  %  | | | | | | | __| '_ \| | | | __|
  %  | |_| | |_| | |_| |_) | |_| | |_ 
  %   \___/ \__,_|\__| .__/ \__,_|\__|
  %                  |_|              
  
%   function K_opt = compute_K_opt(model)
%     % This function computes the local estimation of the global centroid, so where each agent thinks the network centroid is
%     
%     n_models = size(model, 1);
%   
%     K_opt = 0;
%     for j=1:n_models
%       K_opt = K_opt + model{j}.mu*model{j}.K_opt;
%     end
%   end
  function K_opt = compute_K_opt(model)
    % This function computes the local estimation of the global centroid, so where each agent thinks the network centroid is
    
    n_models = size(model, 1);
  
    rho_cp_R2 = 0;
    for j=1:n_models
      rho_cp_R2 = rho_cp_R2 + model{j}.mu*model{j}.rho_cp_R2;
    end

    K_opt = rho_cp_R2;
  end

== matlab function winter_simulink_IMM_control_2states/Torque reference/MATLAB Function2 ==
  data: u input; y output
function y = fcn(u)

y = u(2,:);

== matlab function winter_simulink_IMM_control_2states/Torque reference/Sensor ==
  settings: updateMethod=DISCRETE  sampleTime=simulation.time_step_H
  data: omega input; z output; T_G input; omega_mes output; T_G_mes output; IMM parameter; I_eq parameter; B_eq parameter
function [z, omega_mes, T_G_mes] = sensor(omega, T_G, IMM, I_eq, B_eq)
% This function simulates the measurement o the torque and the generator
% input torque

% Cell
param = cell(6,1);
param{1} = I_eq; % inertia
param{2} = 0; % cp*rho*R^2
param{3} = 0; % K_opt
param{4} = IMM.W; % measure noise
param{5} = IMM.Q; % process noise 
param{6} = B_eq;
% z = zeros(IMM.measure_len, 1);

x = [omega; T_G*1e-6];

z = measurement(x, param, IMM.measure_len);

z(2) =  max(z(2), 1e-6);

omega_mes = z(1);
T_G_mes = z(2);
